simulink library "sfun_storage_heatexchanger"  (R2016b)
settings: Solver=ode45  StartTime=0.0  StopTime=10.0  RelTol=1e-3  EnableMultiTasking=on
settings Model: Creator=drhf  LastModifiedBy=drhf
settings DataIOCC: LimitDataPoints=on  SaveFormat=Array  SignalLoggingSaveFormat=ModelDataLogs
settings OptimizationCC: ExpressionDepthLimit=2147483647  LifeSpan=inf
settings DebuggingCC: UnderspecifiedInitializationDetection=Classic  MergeDetectMultiDrivingBlocksExec=none  SolverPrmCheckMsg=warning  FcnCallInpInsideContextMsg=warning  StateNameClashWarn=warning  SFUnexpectedBacktrackingDiag=warning  SFNoUnconditionalDefaultTransitionDiag=warning  SFExecutionAtInitializationDiag=none
settings HardwareCC: ProdBitPerPointer=32  ProdBitPerSizeT=32  ProdBitPerPtrDiffT=32  ProdLargestAtomicFloat=None  ProdIntDivRoundTo=Undefined  ProdEndianess=Unspecified  ProdWordSize=32  ProdHWDeviceType=32-bit Generic
settings ModelReferenceCC: PropagateSignalLabelsOutOfModel=off
settings GRTTargetCC: TargetLangStandard=C89/C90 (ANSI)  GeneratePreprocessorConditionals=Disable all  CombineOutputUpdateFcns=off  GRTInterface=on
settings ConfigComp: CovMetricSettings=dw  CovHtmlReporting=on  CovSaveCumulativeToWorkspaceVar=on  CovSaveSingleToWorkspaceVar=on  CovExternalEMLEnable=off

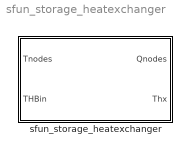
== system sfun_storage_heatexchanger ==
  sfun_storage_heatexchanger : Subsystem  mask(storage heat exchanger){idn=finned tube theoretical  - stratified, nodes=10, inlet=10, outlet=1, p1=0, p2=0, p3=0, p4=0, p5=0, p6=0, p7=0}
      mask prompts: idn "type"; nodes "number of nodes"; inlet "inlet node"; outlet "outlet node"; p1 "Parameter 1"; p2 "Parameter 2"; p3 "Parameter 3"; p4 "Parameter 4"; p5 "Parameter 5"; p6 "Parameter 6"; p7 "Parameter 7"
      mask init:
      | switch(idn)
      |     case 1
      |         id = 201;
      |     case 2
      |         id = 301;
      |     case 3
      |         id = 202;
      |     case 4
      |         id = 302;
      |     case 5
      |         id = 203;
      |     case 6
      |         id = 303;
      |     case 7
      |         id = 204;
      |     case 8
      |         id = 304;
      | end
      mask Help: web(['file:///' fullfile(path_carnot('help'),'StoragePorts_HeatExchangerModels.html')],'-helpbrowser')
      mask TypeOptions idn: smooth tube theoretical | smooth tube theoretical - stratified | finned tube theoretical | finned tube theoretical  - stratified | heat transfer from data fit | heat transfer from data fit  - stratified | heat transfer data fit EN12977 | heat transfer data fit EN12977  - stratified

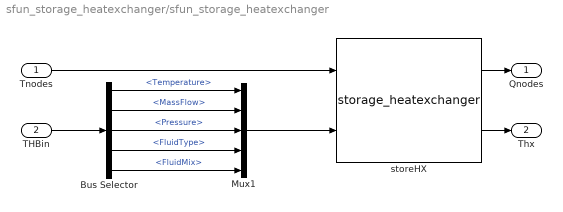
== system sfun_storage_heatexchanger/sfun_storage_heatexchanger ==
  Tnodes : Inport
  THBin : Inport  Port=2
  Bus Selector : BusSelector  OutputSignals=Temperature,MassFlow,Pressure,FluidType,FluidMix
  Mux1 : Mux  Inputs=5
  storeHX : S-Function  FunctionName=storage_heatexchanger  Parameters=id, nodes, inlet, outlet, p1, p2, p3, p4, p5, p6, p7  SFunctionDeploymentMode=off  EnableBusSupport=off  SFcnStateName=DWORK_TS_OLD
      settings: SFcnIsStateOwnerBlock=on
  Qnodes : Outport
  Thx : Outport  Port=2
  wires:
  storeHX/2 -> Thx/1
  THBin/1 -> Bus Selector/1
  storeHX/1 -> Qnodes/1
  Tnodes/1 -> storeHX/1
  Bus Selector/1 -> Mux1/1  "<Temperature>"
  Bus Selector/2 -> Mux1/2  "<MassFlow>"
  Bus Selector/3 -> Mux1/3  "<Pressure>"
  Bus Selector/4 -> Mux1/4  "<FluidType>"
  Bus Selector/5 -> Mux1/5  "<FluidMix>"
  Mux1/1 -> storeHX/2
